simulink model "Overview_of_Control_System"  (R2021a)
settings: Solver=ode45  StartTime=0.0  StopTime=10.0  RelTol=1e-3
settings Model: Creator=sansh  LastModifiedBy=TitusChoi
settings SolverCC: AlgebraicLoopSolver=TrustRegion
settings DataIOCC: ReturnWorkspaceOutputs=off
settings DebuggingCC: SFMachineParentedDataDiag=warning  ArithmeticOperatorsInVariantConditions=warning
settings SFSimCC: SimUseLocalCustomCode=off  CustomCodeUndefinedFunction=UseInterfaceOnly
settings RTWCC: RTWUseLocalCustomCode=off
settings CodeAppCC: StateflowObjectComments=on

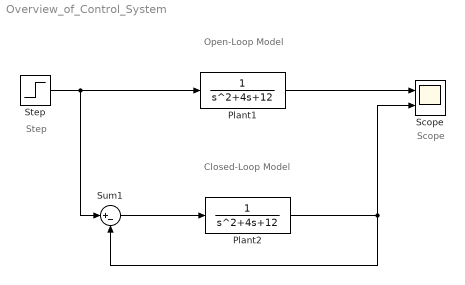
== system Overview_of_Control_System ==
  note: Open-Loop Model
  note: Step
  note: Scope
  note: Closed-Loop Model
  Plant1 : TransferFcn  Denominator=[1 4 12]
  Plant2 : TransferFcn  Denominator=[1 4 12]
  Scope : Scope  NumInputPorts=2
  Step : Step  SampleTime=0
  Sum1 : Sum  Inputs=|+-
  wires:
  Plant1/1 -> Scope/1
  Sum1/1 -> Plant2/1
  Plant2/1 -> Scope/2, Sum1/2
  Step/1 -> Sum1/1, Plant1/1
